simulink model "RC_AVO1"  (Simulink 8.3)
settings: Solver=ode1  StartTime=0.0  StopTime=50  FixedStep=0.01  RelTol=1e-3
settings Model: Creator=Natalia  LastModifiedBy=user
settings DebuggingCC: FcnCallInpInsideContextMsg=UseLocalSettings

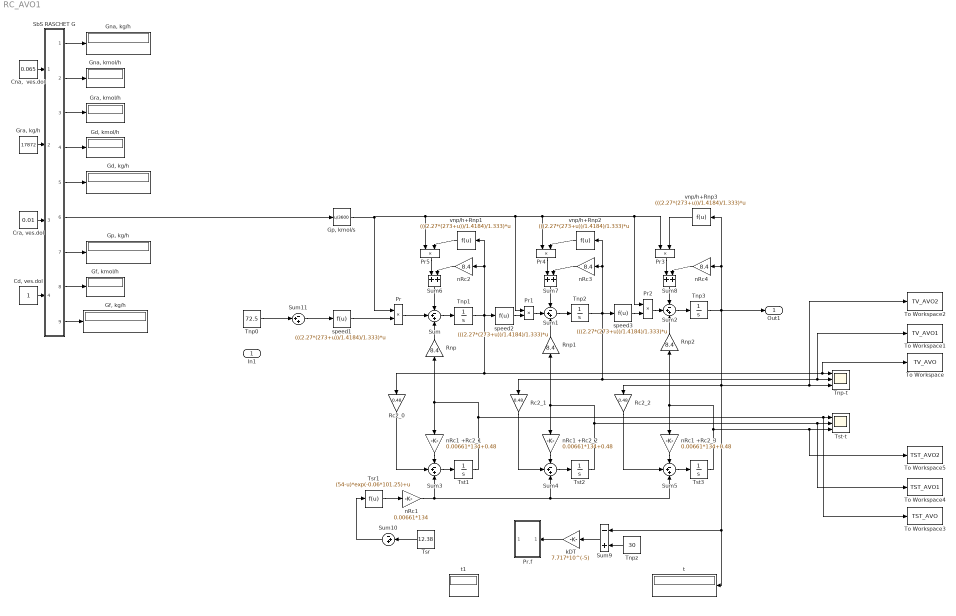
== system RC_AVO1 ==
  In1 : Inport
  "Cd, ves.dol" : Constant
  "Cna,  ves.dol" : Constant  Value=0.065
  "Cra, ves.dol" : Constant  Value=0.01
  "Gd, kg/h" : Display
  "Gd, kmol/h" : Display
  "Gf, kg/h" : Display
  "Gf, kmol/h" : Display
  "Gna, kg/h" : Display
  "Gna, kmol/h" : Display
  "Gp, kmol/s" : Fcn  Expr=u/3600
  "Gp, kg/h" : Display
  "Gra, kg/h" : Constant  Value=17872
  "Gra, kmol/h" : Display
  Pr{,1..5} (6 alike) : Product  RndMeth=Zero
  Pr.f : Subsystem
  Rc2_0 : Gain  Gain=0.48
  Rc2_1 : Gain  Gain=0.48
  Rc2_2 : Gain  Gain=0.48
  Rnp : Gain  Gain=8.4
  Rnp1 : Gain  Gain=8.4
  Rnp2 : Gain  Gain=8.4
  SbS RASCHET G : Subsystem
  Sum{,1..5,10..11} (8 alike) : Sum  Inputs=-++
  Sum6 : Sum
  Sum7 : Sum
  Sum8 : Sum
  Sum9 : Sum  Inputs=-+
  Tnp-t : Scope  NumInputPorts=3
      settings: YMin=67.9728~67.0823~66.2033  YMax=75.1278~74.1435~73.1721
  Tnp0 : Constant  Value=72.5
  Tnp1 : Integrator  InitialCondition=64.99850000
  Tnp2 : Integrator  InitialCondition=57.49700000
  Tnp3 : Integrator  InitialCondition=49.99550000
  Tnpz : Constant  Value=30
  To Workspace : ToWorkspace  VariableName=TV_AVO  SaveFormat=Structure With Time  SampleTime=-1
  To Workspace1 : ToWorkspace  VariableName=TV_AVO1  SaveFormat=Structure With Time  SampleTime=-1
  To Workspace2 : ToWorkspace  VariableName=TV_AVO2  SaveFormat=Structure With Time  SampleTime=-1
  To Workspace3 : ToWorkspace  VariableName=TST_AVO  SaveFormat=Structure With Time  SampleTime=-1
  To Workspace4 : ToWorkspace  VariableName=TST_AVO1  SaveFormat=Structure With Time  SampleTime=-1
  To Workspace5 : ToWorkspace  VariableName=TST_AVO2  SaveFormat=Structure With Time  SampleTime=-1
  Tsr : Constant  Value=12.38
  Tsr1 : Fcn  Expr=(54-u)*exp(-0.06*101.25)+u
  Tst-t : Scope  NumInputPorts=3
      settings: YMin=320.767~573.618~826.668  YMax=354.532~633.998~913.686
  Tst1 : Integrator  InitialCondition=27.020
  Tst2 : Integrator  InitialCondition=25.1550
  Tst3 : Integrator  InitialCondition=23.29
  kDT : Gain  Gain=7.717*10^(-5)
  nRc1 : Gain  Gain=0.00661*134
  nRc1 +Rc2_1 : Gain  Gain=0.00661*134+0.48
  nRc1 +Rc2_2 : Gain  Gain=0.00661*134+0.48
  nRc1 +Rc2_3 : Gain  Gain=0.00661*134+0.48
  nRc2 : Gain  Gain=8.4
  nRc3 : Gain  Gain=8.4
  nRc4 : Gain  Gain=8.4
  speed1 : Fcn  Expr=(((2.27*(273+u))/1.4184)/1.333)*u
  speed2 : Fcn  Expr=(((2.27*(273+u))/1.4184)/1.333)*u
  speed3 : Fcn  Expr=(((2.27*(273+u))/1.4184)/1.333)*u
  t : Display
  t1 : Display
  vnp/h+Rnp1 : Fcn  Expr=(((2.27*(273+u))/1.4184)/1.333)*u
  vnp/h+Rnp2 : Fcn  Expr=(((2.27*(273+u))/1.4184)/1.333)*u
  vnp/h+Rnp3 : Fcn  Expr=(((2.27*(273+u))/1.4184)/1.333)*u
  Out1 : Outport
  wires:
  Sum/1 -> Tnp1/1
  Tnp1/1 -> speed2/1, Rc2_0/1, To Workspace/1, Tnp-t/1, vnp/h+Rnp1/1, nRc2/1
  Sum1/1 -> Tnp2/1
  Tnp2/1 -> speed3/1, Rc2_1/1, To Workspace1/1, Tnp-t/2, vnp/h+Rnp2/1, nRc3/1
  Sum2/1 -> Tnp3/1
  Tnp3/1 -> vnp/h+Rnp3/1, nRc4/1, Out1/1, To Workspace2/1, Tnp-t/3, t/1, Sum9/1, Rc2_2/1
  Rnp1/1 -> Sum1/3
  Rnp2/1 -> Sum2/3
  nRc1 +Rc2_1/1 -> Sum3/1
  Sum3/1 -> Tst1/1
  nRc1 +Rc2_2/1 -> Sum4/1
  Sum4/1 -> Tst2/1
  nRc1 +Rc2_3/1 -> Sum5/1
  Sum5/1 -> Tst3/1
  nRc1/1 -> Sum3/3, Sum4/3, Sum5/3
  Rnp/1 -> Sum/3
  Rc2_1/1 -> Sum4/2
  Rc2_2/1 -> Sum5/2
  Rc2_0/1 -> Sum3/2
  speed1/1 -> Pr/2
  "Gp, kmol/s"/1 -> Pr/1, Pr5/1, Pr1/1, Pr4/1, Pr2/1, Pr3/1
  Pr/1 -> Sum/2
  Pr1/1 -> Sum1/2
  speed2/1 -> Pr1/2
  Pr2/1 -> Sum2/2
  speed3/1 -> Pr2/2
  vnp/h+Rnp3/1 -> Pr3/2
  vnp/h+Rnp2/1 -> Pr4/2
  vnp/h+Rnp1/1 -> Pr5/2
  Pr5/1 -> Sum6/1
  Sum6/1 -> Sum/1
  nRc2/1 -> Sum6/2
  nRc3/1 -> Sum7/2
  Pr4/1 -> Sum7/1
  Sum7/1 -> Sum1/1
  nRc4/1 -> Sum8/2
  Pr3/1 -> Sum8/1
  Sum8/1 -> Sum2/1
  "Cna,  ves.dol"/1 -> SbS RASCHET G/1(In1)
  "Cra, ves.dol"/1 -> SbS RASCHET G/3(In3)
  "Cd, ves.dol"/1 -> SbS RASCHET G/4(In4)
  "Gra, kg/h"/1 -> SbS RASCHET G/2(In2)
  SbS RASCHET G/1(Out1) -> "Gna, kg/h"/1
  SbS RASCHET G/5(Out5) -> "Gd, kg/h"/1
  SbS RASCHET G/7(Out7) -> "Gp, kg/h"/1
  SbS RASCHET G/9(Out9) -> "Gf, kg/h"/1
  SbS RASCHET G/2(Out2) -> "Gna, kmol/h"/1
  SbS RASCHET G/3(Out3) -> "Gra, kmol/h"/1
  SbS RASCHET G/4(Out4) -> "Gd, kmol/h"/1
  SbS RASCHET G/6(Out6) -> "Gp, kmol/s"/1
  SbS RASCHET G/8(Out8) -> "Gf, kmol/h"/1
  Sum9/1 -> kDT/1
  Tnpz/1 -> Sum9/2
  kDT/1 -> Pr.f/1(In1)
  Tsr1/1 -> nRc1/1
  Sum10/1 -> Tsr1/1
  Tst1/1 -> nRc1 +Rc2_1/1, Rnp/1, Tst-t/1, To Workspace3/1
  Tst2/1 -> nRc1 +Rc2_2/1, Rnp1/1, To Workspace4/1, Tst-t/2
  Tst3/1 -> nRc1 +Rc2_3/1, Rnp2/1, To Workspace5/1, Tst-t/3
  Sum11/1 -> speed1/1
  Tnp0/1 -> Sum11/2
  Tsr/1 -> Sum10/2

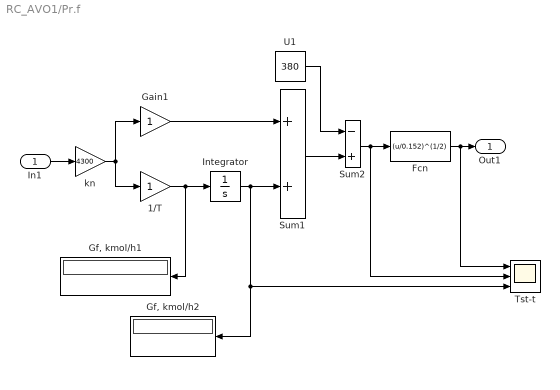
== system RC_AVO1/Pr.f ==
  In1 : Inport
  1/T : Gain
  Fcn : Fcn  Expr=(u/0.152)^(1/2)
  Gain1 : Gain
  "Gf, kmol/h1" : Display
  "Gf, kmol/h2" : Display
  Integrator : Integrator  InitialCondition=403.6
  Sum1 : Sum
  Sum2 : Sum  Inputs=-+
  Tst-t : Scope  NumInputPorts=3
      settings: YMin=320.767~573.618~826.668  YMax=354.532~633.998~913.686  SaveName=ScopeData2
  U1 : Constant  Value=380
  kn : Gain  Gain=4300
  Out1 : Outport
  wires:
  kn/1 -> 1/T/1, Gain1/1
  1/T/1 -> Integrator/1, "Gf, kmol/h1"/1
  Integrator/1 -> Sum1/2, Tst-t/3, "Gf, kmol/h2"/1
  Gain1/1 -> Sum1/1
  Sum1/1 -> Sum2/2
  U1/1 -> Sum2/1
  In1/1 -> kn/1
  Fcn/1 -> Tst-t/1, Out1/1
  Sum2/1 -> Tst-t/2, Fcn/1

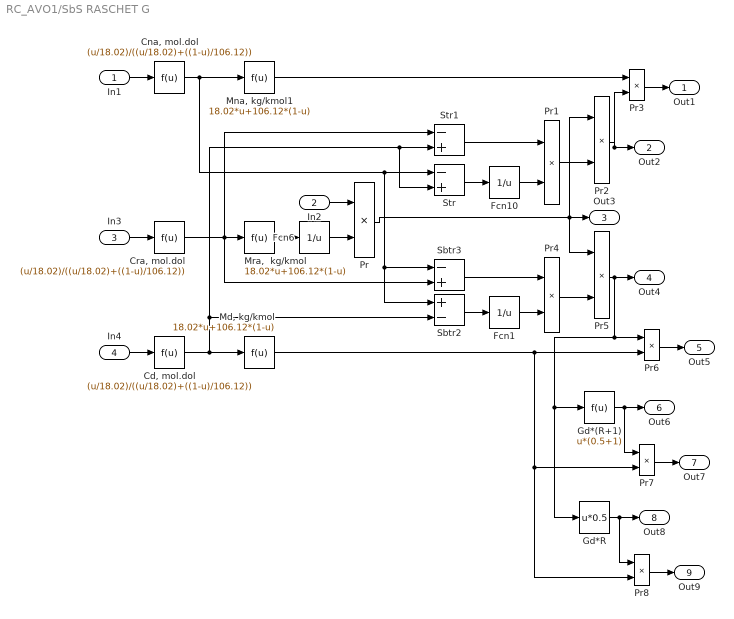
== system RC_AVO1/SbS RASCHET G ==
  In1 : Inport
  In2 : Inport  Port=2
  In3 : Inport  Port=3
  In4 : Inport  Port=4
  "Cd, mol.dol" : Fcn  Expr=(u/18.02)/((u/18.02)+((1-u)/106.12))
  "Cna, mol.dol" : Fcn  Expr=(u/18.02)/((u/18.02)+((1-u)/106.12))
  "Cra, mol.dol" : Fcn  Expr=(u/18.02)/((u/18.02)+((1-u)/106.12))
  Fcn1 : Fcn  Expr=1/u
  Fcn10 : Fcn  Expr=1/u
  Fcn6 : Fcn  Expr=1/u
  Gd*(R+1) : Fcn  Expr=u*(0.5+1)
  Gd*R : Fcn  Expr=u*0.5
  "Md, kg/kmol" : Fcn  Expr=18.02*u+106.12*(1-u)
  "Mna, kg/kmol1" : Fcn  Expr=18.02*u+106.12*(1-u)
  "Mra,  kg/kmol" : Fcn  Expr=18.02*u+106.12*(1-u)
  Pr{,1..8} (9 alike) : Product  RndMeth=Zero
  Sbtr2 : Sum  Inputs=+-
  Sbtr3 : Sum  Inputs=-+
  Str : Sum  Inputs=-+
  Str1 : Sum  Inputs=-+
  Out1 : Outport
  Out2 : Outport  Port=2
  Out3 : Outport  Port=3
  Out4 : Outport  Port=4
  Out5 : Outport  Port=5
  Out6 : Outport  Port=6
  Out7 : Outport  Port=7
  Out8 : Outport  Port=8
  Out9 : Outport  Port=9
  wires:
  "Mna, kg/kmol1"/1 -> Pr3/1
  "Cna, mol.dol"/1 -> "Mna, kg/kmol1"/1, Str/1, Sbtr3/1, Sbtr2/1
  "Cra, mol.dol"/1 -> "Mra,  kg/kmol"/1, Str1/1, Sbtr3/2
  "Cd, mol.dol"/1 -> "Md, kg/kmol"/1, Str1/2, Str/2, Sbtr2/2
  "Mra,  kg/kmol"/1 -> Fcn6/1
  Fcn6/1 -> Pr/2
  Pr/1 -> Pr2/1, Out3/1, Pr5/1
  Str/1 -> Fcn10/1
  Fcn10/1 -> Pr1/2
  Pr2/1 -> Pr3/2, Out2/1
  Pr1/1 -> Pr2/2
  Str1/1 -> Pr1/1
  Fcn1/1 -> Pr4/2
  Pr5/1 -> Pr6/1, Gd*(R+1)/1, Gd*R/1, Out4/1
  Pr4/1 -> Pr5/2
  "Md, kg/kmol"/1 -> Pr6/2, Pr7/2, Pr8/2
  Sbtr2/1 -> Fcn1/1
  Sbtr3/1 -> Pr4/1
  Gd*(R+1)/1 -> Pr7/1, Out6/1
  Gd*R/1 -> Pr8/1, Out8/1
  In1/1 -> "Cna, mol.dol"/1
  Pr3/1 -> Out1/1
  In2/1 -> Pr/1
  In3/1 -> "Cra, mol.dol"/1
  Pr6/1 -> Out5/1
  In4/1 -> "Cd, mol.dol"/1
  Pr7/1 -> Out7/1
  Pr8/1 -> Out9/1
